simulink model "Simulink"  (R2025a)
settings: Solver=FixedStepDiscrete  StartTime=0.0  StopTime=80  FixedStep=1  RelTol=1e-3
libraries: simulink_extras x14
settings Model: SnapshotBufferSize=35  PacingRate=2  Creator=dell  LastModifiedBy=LENOVO

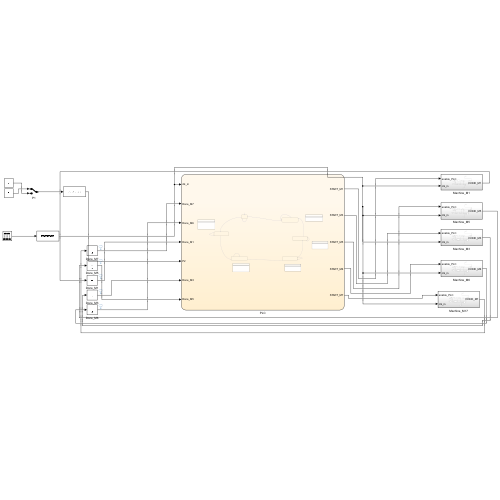
[thumbnail: Simulink's stored preview of the top-level diagram]
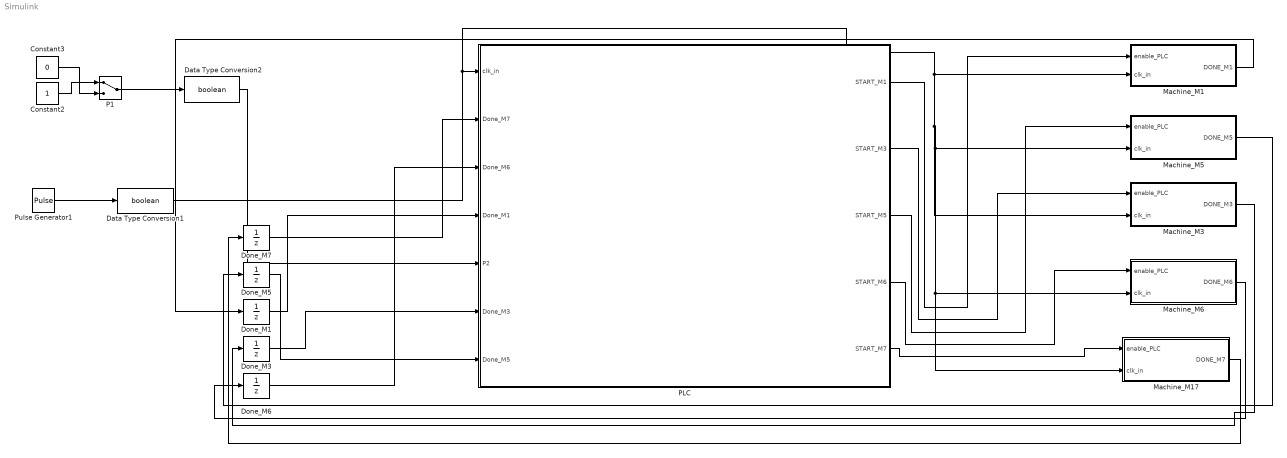
== system Simulink ==
  Constant2 : Constant  OutDataTypeStr=boolean
  Constant3 : Constant  Value=0  OutDataTypeStr=boolean
  Data Type Conversion1 : DataTypeConversion  OutDataTypeStr=boolean  SaturateOnIntegerOverflow=off  RndMeth=Floor
  Data Type Conversion2 : DataTypeConversion  OutDataTypeStr=boolean  SaturateOnIntegerOverflow=off  RndMeth=Floor
  Done_M{1,3,5..7} (5 alike) : UnitDelay  HasFrameUpgradeWarning=on
  Machine_M1 : Subsystem
  Machine_M17 : Subsystem
  Machine_M3 : Subsystem
  Machine_M5 : Subsystem
  Machine_M6 : Subsystem
  P1 : ManualSwitch
  PLC : Stateflow chart  TreatAsAtomicUnit=on
      settings: PortSchema="{\"entries\":[{\"content\":{\"sides\":[{\"content\":{\"connectorIds\":[\"In1\",\"In2\",\"In5\",\"In6\",\"In7\",\"In4\",\"In3\"]},\"type\":\"ConnectorPlacement.EquallySpacedRectSide\",\"uuid\":\"17f713a5-d983-479c-9e5e-6bf6c33331de\"},{\"content\":{\"connectorIds\":[\"Out1\",\"Out5\",\"Out2\",\"Out4\",\"Out3\"],\"side\":\"RIGHT\"},\"type\":\"ConnectorPlacement.EquallySpacedRectSide\",\"uuid\":\"d38a5cd9-5070-4c28-a52d-34bc8e7c4c10\"},{\"content\":{\"side\":\"TOP\"},\"type\":\"ConnectorPlacement.EquallySpacedRectSide\",\"uuid\":\"4971cf38-fc56-403e-81e2-f618dbc9148e\"}]},\"type\":\"ConnectorPlacement.EquallySpacedConnector\",\"uuid\":\"d5f3cc63-d87c-4b36-b9e3-2569f685359e\"}],\"packageUris\":[\"http://schema.mathworks.com/mf0/Connector/R2020b\"],\"version\":\"1.0\"}"
  Pulse Generator1 : DiscretePulseGenerator
  wires:
  Pulse Generator1/1 -> Data Type Conversion1/1
  Data Type Conversion1/1 -> Machine_M3/2(clk_in), Machine_M17/2(clk_in), Machine_M6/2(clk_in), Machine_M5/2(clk_in), Machine_M1/2(clk_in), PLC/1(clk_in)
  Constant3/1 -> P1/2
  Constant2/1 -> P1/1
  P1/1 -> Data Type Conversion2/1
  Done_M7/1 -> PLC/2(Done_M7)
  Done_M5/1 -> PLC/3(Done_M5)
  Done_M3/1 -> PLC/4(Done_M3)
  Done_M6/1 -> PLC/5(Done_M6)
  PLC/1(START_M1) -> Machine_M1/1(enable_PLC)
  PLC/2(START_M5) -> Machine_M5/1(enable_PLC)
  PLC/3(START_M7) -> Machine_M17/1(enable_PLC)
  PLC/4(START_M6) -> Machine_M6/1(enable_PLC)
  PLC/5(START_M3) -> Machine_M3/1(enable_PLC)
  Machine_M1/1(DONE_M1) -> Done_M1/1
  Machine_M5/1(DONE_M5) -> Done_M5/1
  Machine_M3/1(DONE_M3) -> Done_M3/1
  Machine_M6/1(DONE_M6) -> Done_M6/1
  Machine_M17/1(DONE_M7) -> Done_M7/1
  Done_M1/1 -> PLC/6(Done_M1)
  Data Type Conversion2/1 -> PLC/7(P2)

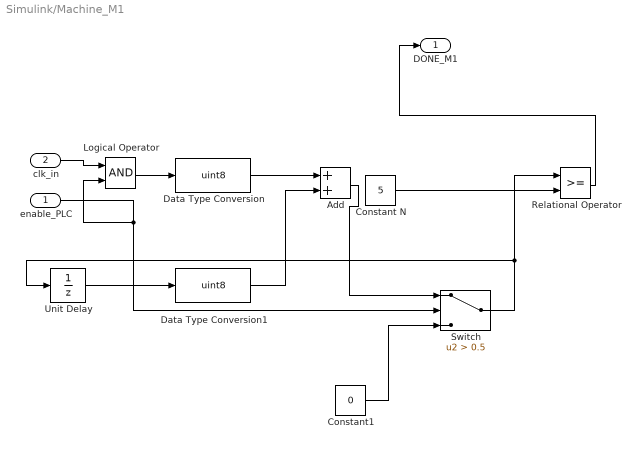
== system Simulink/Machine_M1 ==
  enable_PLC : Inport
  clk_in : Inport  Port=2
  Add : Sum
  Constant N : Constant  Value=5  OutDataTypeStr=uint8
  Constant1 : Constant  Value=0
  Data Type Conversion : DataTypeConversion  OutDataTypeStr=uint8  SaturateOnIntegerOverflow=off  RndMeth=Floor
  Data Type Conversion1 : DataTypeConversion  OutDataTypeStr=uint8  SaturateOnIntegerOverflow=off  RndMeth=Floor
  Logical Operator : Logic  AllPortsSameDT=off  OutDataTypeStr=boolean
  Relational Operator : RelationalOperator  OutDataTypeStr=boolean  RndMeth=Simplest  InputSameDT=off
  Switch : Switch  Criteria=u2 > Threshold  Threshold=0.5  SaturateOnIntegerOverflow=off  InputSameDT=off
  Unit Delay : UnitDelay  HasFrameUpgradeWarning=on
  DONE_M1 : Outport
  wires:
  Constant1/1 -> Switch/3
  Constant N/1 -> Relational Operator/2
  Relational Operator/1 -> DONE_M1/1
  clk_in/1 -> Logical Operator/1
  enable_PLC/1 -> Switch/2, Logical Operator/2
  Logical Operator/1 -> Data Type Conversion/1
  Unit Delay/1 -> Data Type Conversion1/1
  Add/1 -> Switch/1
  Switch/1 -> Relational Operator/1, Unit Delay/1
  Data Type Conversion/1 -> Add/1
  Data Type Conversion1/1 -> Add/2

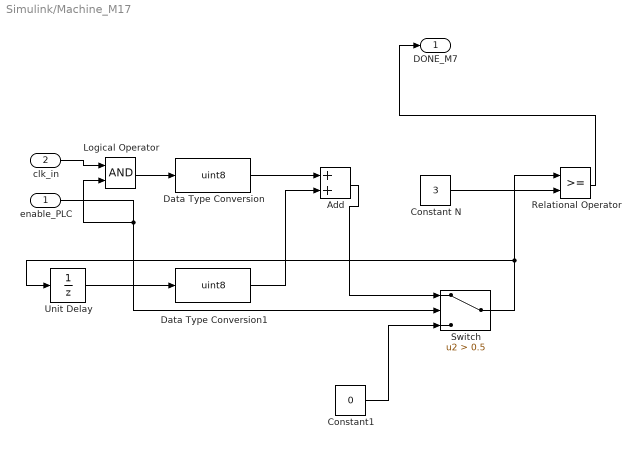
== system Simulink/Machine_M17 ==
  enable_PLC : Inport
  clk_in : Inport  Port=2
  Add : Sum
  Constant N : Constant  Value=3  OutDataTypeStr=uint8
  Constant1 : Constant  Value=0
  Data Type Conversion : DataTypeConversion  OutDataTypeStr=uint8  SaturateOnIntegerOverflow=off  RndMeth=Floor
  Data Type Conversion1 : DataTypeConversion  OutDataTypeStr=uint8  SaturateOnIntegerOverflow=off  RndMeth=Floor
  Logical Operator : Logic  AllPortsSameDT=off  OutDataTypeStr=boolean
  Relational Operator : RelationalOperator  OutDataTypeStr=boolean  RndMeth=Simplest  InputSameDT=off
  Switch : Switch  Criteria=u2 > Threshold  Threshold=0.5  SaturateOnIntegerOverflow=off  InputSameDT=off
  Unit Delay : UnitDelay  HasFrameUpgradeWarning=on
  DONE_M7 : Outport
  wires:
  Constant1/1 -> Switch/3
  Switch/1 -> Relational Operator/1, Unit Delay/1
  enable_PLC/1 -> Switch/2, Logical Operator/2
  Logical Operator/1 -> Data Type Conversion/1
  Constant N/1 -> Relational Operator/2
  clk_in/1 -> Logical Operator/1
  Data Type Conversion/1 -> Add/1
  Data Type Conversion1/1 -> Add/2
  Add/1 -> Switch/1
  Unit Delay/1 -> Data Type Conversion1/1
  Relational Operator/1 -> DONE_M7/1

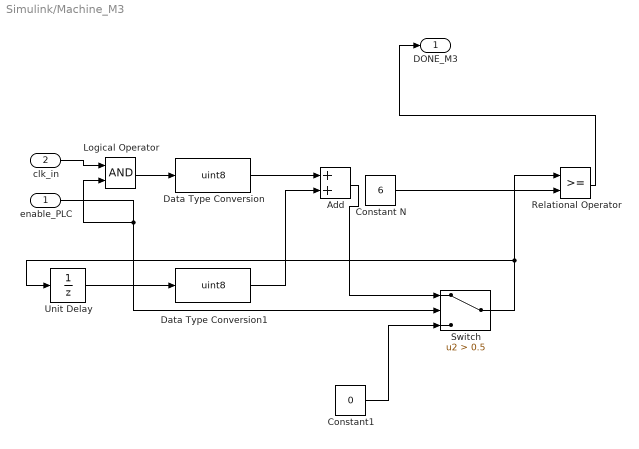
== system Simulink/Machine_M3 ==
  enable_PLC : Inport
  clk_in : Inport  Port=2
  Add : Sum
  Constant N : Constant  Value=6  OutDataTypeStr=uint8
  Constant1 : Constant  Value=0
  Data Type Conversion : DataTypeConversion  OutDataTypeStr=uint8  SaturateOnIntegerOverflow=off  RndMeth=Floor
  Data Type Conversion1 : DataTypeConversion  OutDataTypeStr=uint8  SaturateOnIntegerOverflow=off  RndMeth=Floor
  Logical Operator : Logic  AllPortsSameDT=off  OutDataTypeStr=boolean
  Relational Operator : RelationalOperator  OutDataTypeStr=boolean  RndMeth=Simplest  InputSameDT=off
  Switch : Switch  Criteria=u2 > Threshold  Threshold=0.5  SaturateOnIntegerOverflow=off  InputSameDT=off
  Unit Delay : UnitDelay  HasFrameUpgradeWarning=on
  DONE_M3 : Outport
  wires:
  Constant1/1 -> Switch/3
  Switch/1 -> Relational Operator/1, Unit Delay/1
  enable_PLC/1 -> Switch/2, Logical Operator/2
  Logical Operator/1 -> Data Type Conversion/1
  Constant N/1 -> Relational Operator/2
  clk_in/1 -> Logical Operator/1
  Data Type Conversion/1 -> Add/1
  Data Type Conversion1/1 -> Add/2
  Add/1 -> Switch/1
  Unit Delay/1 -> Data Type Conversion1/1
  Relational Operator/1 -> DONE_M3/1

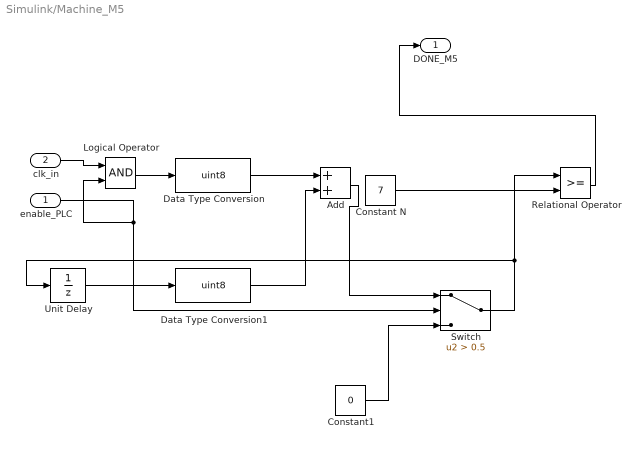
== system Simulink/Machine_M5 ==
  enable_PLC : Inport
  clk_in : Inport  Port=2
  Add : Sum
  Constant N : Constant  Value=7  OutDataTypeStr=uint8
  Constant1 : Constant  Value=0
  Data Type Conversion : DataTypeConversion  OutDataTypeStr=uint8  SaturateOnIntegerOverflow=off  RndMeth=Floor
  Data Type Conversion1 : DataTypeConversion  OutDataTypeStr=uint8  SaturateOnIntegerOverflow=off  RndMeth=Floor
  Logical Operator : Logic  AllPortsSameDT=off  OutDataTypeStr=boolean
  Relational Operator : RelationalOperator  OutDataTypeStr=boolean  RndMeth=Simplest  InputSameDT=off
  Switch : Switch  Criteria=u2 > Threshold  Threshold=0.5  SaturateOnIntegerOverflow=off  InputSameDT=off
  Unit Delay : UnitDelay  HasFrameUpgradeWarning=on
  DONE_M5 : Outport
  wires:
  Constant1/1 -> Switch/3
  Switch/1 -> Relational Operator/1, Unit Delay/1
  enable_PLC/1 -> Switch/2, Logical Operator/2
  Logical Operator/1 -> Data Type Conversion/1
  Constant N/1 -> Relational Operator/2
  clk_in/1 -> Logical Operator/1
  Data Type Conversion/1 -> Add/1
  Data Type Conversion1/1 -> Add/2
  Add/1 -> Switch/1
  Unit Delay/1 -> Data Type Conversion1/1
  Relational Operator/1 -> DONE_M5/1

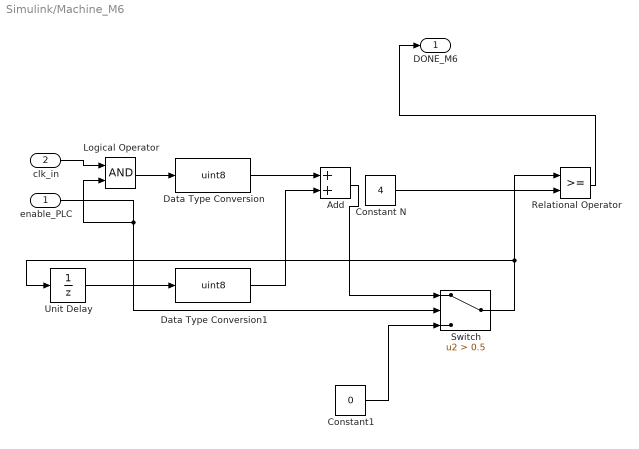
== system Simulink/Machine_M6 ==
  enable_PLC : Inport
  clk_in : Inport  Port=2
  Add : Sum
  Constant N : Constant  Value=4  OutDataTypeStr=uint8
  Constant1 : Constant  Value=0
  Data Type Conversion : DataTypeConversion  OutDataTypeStr=uint8  SaturateOnIntegerOverflow=off  RndMeth=Floor
  Data Type Conversion1 : DataTypeConversion  OutDataTypeStr=uint8  SaturateOnIntegerOverflow=off  RndMeth=Floor
  Logical Operator : Logic  AllPortsSameDT=off  OutDataTypeStr=boolean
  Relational Operator : RelationalOperator  OutDataTypeStr=boolean  RndMeth=Simplest  InputSameDT=off
  Switch : Switch  Criteria=u2 > Threshold  Threshold=0.5  SaturateOnIntegerOverflow=off  InputSameDT=off
  Unit Delay : UnitDelay  HasFrameUpgradeWarning=on
  DONE_M6 : Outport
  wires:
  Constant1/1 -> Switch/3
  Switch/1 -> Relational Operator/1, Unit Delay/1
  enable_PLC/1 -> Switch/2, Logical Operator/2
  Logical Operator/1 -> Data Type Conversion/1
  Constant N/1 -> Relational Operator/2
  clk_in/1 -> Logical Operator/1
  Data Type Conversion/1 -> Add/1
  Data Type Conversion1/1 -> Add/2
  Add/1 -> Switch/1
  Unit Delay/1 -> Data Type Conversion1/1
  Relational Operator/1 -> DONE_M6/1

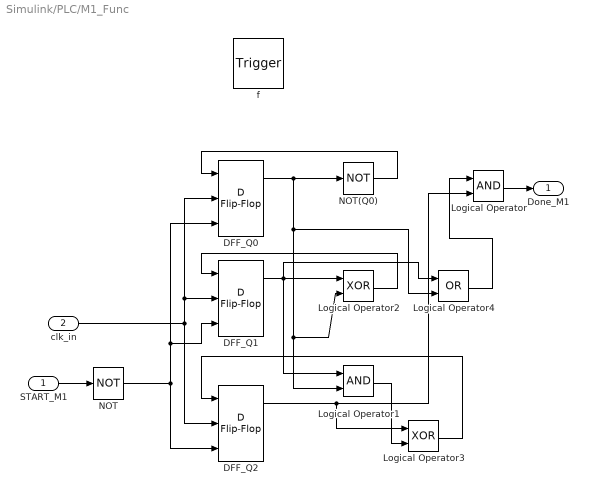
== system Simulink/PLC/M1_Func ==
  START_M1 : Inport  OutDataTypeStr=double  PortDimensions=1
  clk_in : Inport  Port=2  OutDataTypeStr=double  PortDimensions=1
  f : TriggerPort  TriggerType=function-call  VariantControl=(inherit)
      settings: CopyFcn=Stateflow.SLINSF.SimulinkMan.removeBlockPreDeleteFcn  PreDeleteFcn=Stateflow.SLINSF.SimulinkMan.unsafePredeleteFcn
  DFF_Q0 : simulink_extras/Flip Flops/D Flip-Flop
  DFF_Q1 : simulink_extras/Flip Flops/D Flip-Flop
  DFF_Q2 : simulink_extras/Flip Flops/D Flip-Flop
  Logical Operator : Logic  AllPortsSameDT=off  OutDataTypeStr=boolean
  Logical Operator1 : Logic  AllPortsSameDT=off  OutDataTypeStr=boolean
  Logical Operator2 : Logic  Operator=XOR  AllPortsSameDT=off  OutDataTypeStr=boolean
  Logical Operator3 : Logic  Operator=XOR  AllPortsSameDT=off  OutDataTypeStr=boolean
  Logical Operator4 : Logic  Operator=OR  AllPortsSameDT=off  OutDataTypeStr=boolean
  NOT : Logic  Operator=NOT  IconShape=distinctive  AllPortsSameDT=off  OutDataTypeStr=boolean
  NOT(Q0) : Logic  Operator=NOT  IconShape=distinctive  AllPortsSameDT=off  OutDataTypeStr=boolean
  Done_M1 : Outport  OutDataTypeStr=boolean  PortDimensions=1
  wires:
  START_M1/1 -> NOT/1
  NOT/1 -> DFF_Q0/3, DFF_Q1/3, DFF_Q2/3
  clk_in/1 -> DFF_Q0/2, DFF_Q1/2, DFF_Q2/2
  DFF_Q0/1 -> Logical Operator4/2, Logical Operator1/2, Logical Operator2/2, NOT(Q0)/1
  DFF_Q1/1 -> Logical Operator4/1, Logical Operator1/1, Logical Operator2/1
  DFF_Q2/1 -> Logical Operator/2, Logical Operator3/1
  Logical Operator1/1 -> Logical Operator3/2
  NOT(Q0)/1 -> DFF_Q0/1
  Logical Operator2/1 -> DFF_Q1/1
  Logical Operator3/1 -> DFF_Q2/1
  Logical Operator/1 -> Done_M1/1
  Logical Operator4/1 -> Logical Operator/1

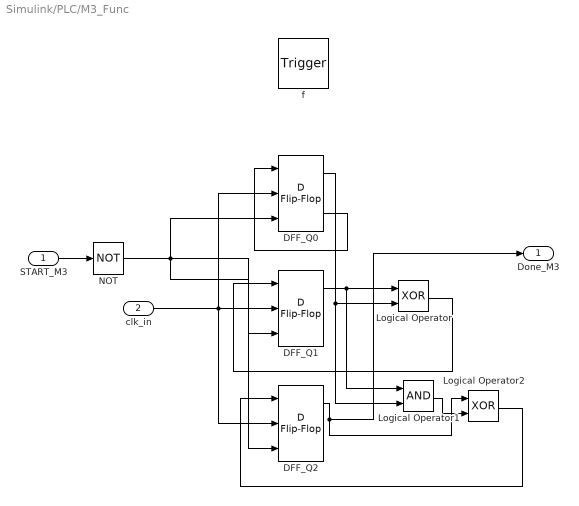
== system Simulink/PLC/M3_Func ==
  START_M3 : Inport  OutDataTypeStr=boolean  PortDimensions=1
  clk_in : Inport  Port=2  OutDataTypeStr=boolean  PortDimensions=1
  f : TriggerPort  TriggerType=function-call  VariantControl=(inherit)
      settings: CopyFcn=Stateflow.SLINSF.SimulinkMan.removeBlockPreDeleteFcn  PreDeleteFcn=Stateflow.SLINSF.SimulinkMan.unsafePredeleteFcn
  DFF_Q0 : simulink_extras/Flip Flops/D Flip-Flop
  DFF_Q1 : simulink_extras/Flip Flops/D Flip-Flop
  DFF_Q2 : simulink_extras/Flip Flops/D Flip-Flop
  Logical Operator : Logic  Operator=XOR  AllPortsSameDT=off  OutDataTypeStr=boolean
  Logical Operator1 : Logic  AllPortsSameDT=off  OutDataTypeStr=boolean
  Logical Operator2 : Logic  Operator=XOR  AllPortsSameDT=off  OutDataTypeStr=boolean
  NOT : Logic  Operator=NOT  IconShape=distinctive  AllPortsSameDT=off  OutDataTypeStr=boolean
  Done_M3 : Outport  OutDataTypeStr=boolean  PortDimensions=1
  wires:
  clk_in/1 -> DFF_Q2/2, DFF_Q1/2, DFF_Q0/2
  START_M3/1 -> NOT/1
  NOT/1 -> DFF_Q2/3, DFF_Q1/3, DFF_Q0/3
  DFF_Q0/2 -> DFF_Q0/1
  DFF_Q1/1 -> Logical Operator1/1, Logical Operator/1
  DFF_Q0/1 -> Logical Operator1/2, Logical Operator/2
  Logical Operator/1 -> DFF_Q1/1
  DFF_Q2/1 -> Done_M3/1, Logical Operator2/1
  Logical Operator1/1 -> Logical Operator2/2
  Logical Operator2/1 -> DFF_Q2/1

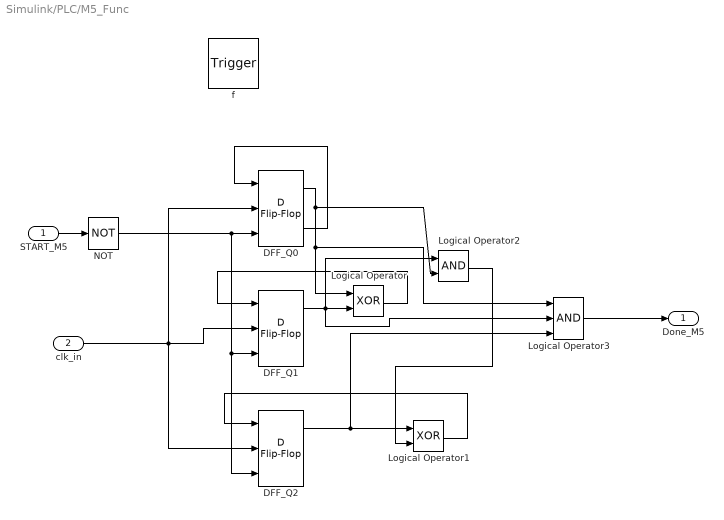
== system Simulink/PLC/M5_Func ==
  START_M5 : Inport  OutDataTypeStr=boolean  PortDimensions=1
  clk_in : Inport  Port=2  OutDataTypeStr=boolean  PortDimensions=1
  f : TriggerPort  TriggerType=function-call  VariantControl=(inherit)
      settings: CopyFcn=Stateflow.SLINSF.SimulinkMan.removeBlockPreDeleteFcn  PreDeleteFcn=Stateflow.SLINSF.SimulinkMan.unsafePredeleteFcn
  DFF_Q0 : simulink_extras/Flip Flops/D Flip-Flop
  DFF_Q1 : simulink_extras/Flip Flops/D Flip-Flop
  DFF_Q2 : simulink_extras/Flip Flops/D Flip-Flop
  Logical Operator : Logic  Operator=XOR  AllPortsSameDT=off  OutDataTypeStr=boolean
  Logical Operator1 : Logic  Operator=XOR  AllPortsSameDT=off  OutDataTypeStr=boolean
  Logical Operator2 : Logic  AllPortsSameDT=off  OutDataTypeStr=boolean
  Logical Operator3 : Logic  Inputs=3  AllPortsSameDT=off  OutDataTypeStr=boolean
  NOT : Logic  Operator=NOT  IconShape=distinctive  AllPortsSameDT=off  OutDataTypeStr=boolean
  Done_M5 : Outport  OutDataTypeStr=boolean  PortDimensions=1
  wires:
  clk_in/1 -> DFF_Q2/2, DFF_Q0/2, DFF_Q1/2
  START_M5/1 -> NOT/1
  NOT/1 -> DFF_Q2/3, DFF_Q1/3, DFF_Q0/3
  DFF_Q0/2 -> DFF_Q0/1
  DFF_Q1/1 -> Logical Operator3/2, Logical Operator2/1, Logical Operator/2
  DFF_Q0/1 -> Logical Operator2/2, Logical Operator3/1, Logical Operator/1
  Logical Operator/1 -> DFF_Q1/1
  Logical Operator2/1 -> Logical Operator1/2
  DFF_Q2/1 -> Logical Operator3/3, Logical Operator1/1
  Logical Operator1/1 -> DFF_Q2/1
  Logical Operator3/1 -> Done_M5/1

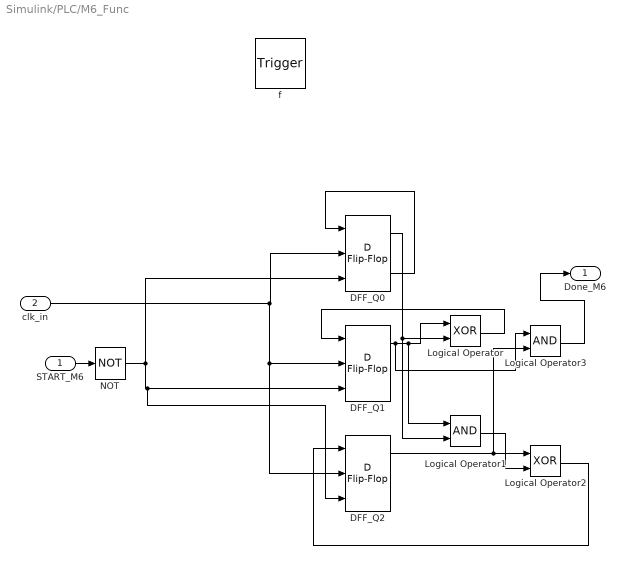
== system Simulink/PLC/M6_Func ==
  START_M6 : Inport  OutDataTypeStr=boolean  PortDimensions=1
  clk_in : Inport  Port=2  OutDataTypeStr=boolean  PortDimensions=1
  f : TriggerPort  TriggerType=function-call  VariantControl=(inherit)
      settings: CopyFcn=Stateflow.SLINSF.SimulinkMan.removeBlockPreDeleteFcn  PreDeleteFcn=Stateflow.SLINSF.SimulinkMan.unsafePredeleteFcn
  DFF_Q0 : simulink_extras/Flip Flops/D Flip-Flop
  DFF_Q1 : simulink_extras/Flip Flops/D Flip-Flop
  DFF_Q2 : simulink_extras/Flip Flops/D Flip-Flop
  Logical Operator : Logic  Operator=XOR  AllPortsSameDT=off  OutDataTypeStr=boolean
  Logical Operator1 : Logic  AllPortsSameDT=off  OutDataTypeStr=boolean
  Logical Operator2 : Logic  Operator=XOR  AllPortsSameDT=off  OutDataTypeStr=boolean
  Logical Operator3 : Logic  AllPortsSameDT=off  OutDataTypeStr=boolean
  NOT : Logic  Operator=NOT  IconShape=distinctive  AllPortsSameDT=off  OutDataTypeStr=boolean
  Done_M6 : Outport  OutDataTypeStr=boolean  PortDimensions=1
  wires:
  clk_in/1 -> DFF_Q2/2, DFF_Q1/2, DFF_Q0/2
  START_M6/1 -> NOT/1
  NOT/1 -> DFF_Q0/3, DFF_Q2/3, DFF_Q1/3
  DFF_Q0/2 -> DFF_Q0/1
  DFF_Q1/1 -> Logical Operator3/1, Logical Operator1/1, Logical Operator/1
  DFF_Q0/1 -> Logical Operator1/2, Logical Operator/2
  Logical Operator/1 -> DFF_Q1/1
  Logical Operator1/1 -> Logical Operator2/2
  DFF_Q2/1 -> Logical Operator3/2, Logical Operator2/1
  Logical Operator2/1 -> DFF_Q2/1
  Logical Operator3/1 -> Done_M6/1

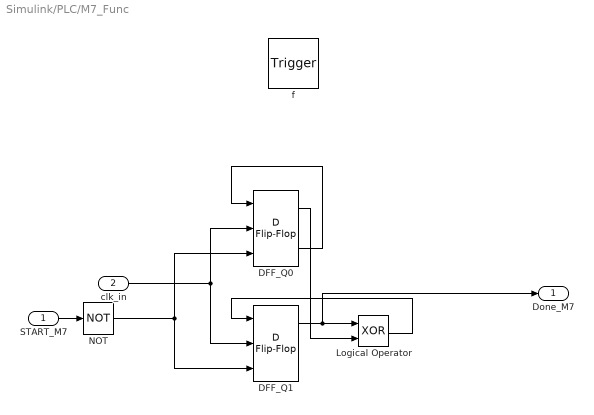
== system Simulink/PLC/M7_Func ==
  START_M7 : Inport  OutDataTypeStr=boolean  PortDimensions=1
  clk_in : Inport  Port=2  OutDataTypeStr=boolean  PortDimensions=1
  f : TriggerPort  TriggerType=function-call  VariantControl=(inherit)
      settings: CopyFcn=Stateflow.SLINSF.SimulinkMan.removeBlockPreDeleteFcn  PreDeleteFcn=Stateflow.SLINSF.SimulinkMan.unsafePredeleteFcn
  DFF_Q0 : simulink_extras/Flip Flops/D Flip-Flop
  DFF_Q1 : simulink_extras/Flip Flops/D Flip-Flop
  Logical Operator : Logic  Operator=XOR  AllPortsSameDT=off  OutDataTypeStr=boolean
  NOT : Logic  Operator=NOT  IconShape=distinctive  AllPortsSameDT=off  OutDataTypeStr=boolean
  Done_M7 : Outport  OutDataTypeStr=boolean  PortDimensions=1
  wires:
  clk_in/1 -> DFF_Q0/2, DFF_Q1/2
  START_M7/1 -> NOT/1
  NOT/1 -> DFF_Q0/3, DFF_Q1/3
  DFF_Q0/2 -> DFF_Q0/1
  DFF_Q1/1 -> Done_M7/1, Logical Operator/1
  DFF_Q0/1 -> Logical Operator/2
  Logical Operator/1 -> DFF_Q1/1

== stateflow chart Simulink/PLC ==
  settings: sampleTime=2
  state IDLE
  state Done_M7 = M7_Func(START_M7,clk_in) [function]
  state M7
    START_M7=true;
  state Done_M1 = M1_Func(START_M1,clk_in) [function]
  state M1
    START_M1=true;
  state M6
    START_M6= true;
  state Done_M6 = M6_Func(START_M6,clk_in) [function]
  state M5
    START_M5=true;
  state M3
    START_M3=true;
  state Done_M5 = M5_Func(START_M5,clk_in) [function]
  state Done_M3 = M3_Func(START_M3,clk_in) [function]
  (default) -> IDLE
  M7 -> M7 [order 1] : [Done_M7==0]
  M7 -> IDLE [order 2] : [Done_M7==1]
  IDLE -> M1 [order 1] : [P2==1]
  M6 -> M7 [order 1] : [Done_M6==1]
  IDLE -> IDLE [order 2] : [P2==0]
  M1 -> M1 [order 2] : [Done_M1==0]
  M1 -> M5 [order 1] : [Done_M1==1]
  M6 -> M6 [order 2] : [Done_M6==0]
  M3 -> M6 [order 1] : [Done_M3==1]
  M5 -> M5 [order 2] : [Done_M5==0]
  M3 -> M3 [order 2] : [Done_M3==0]
  M5 -> M3 [order 1] : [Done_M5==1]
  data: START_M7 function_input boolean size=1; Done_M7 function_output boolean size=1; clk_in function_input boolean size=1; Done_M1 function_output boolean size=1; START_M1 function_input double size=1; clk_in function_input double size=1; START_M6 function_input boolean size=1; Done_M6 function_output boolean size=1; clk_in function_input boolean size=1; START_M5 function_input boolean size=1; Done_M5 function_output boolean size=1; clk_in function_input boolean size=1; START_M3 function_input boolean size=1; Done_M3 function_output boolean size=1; clk_in function_input boolean size=1; clk_in input; START_M1 output boolean size=1; START_M5 output boolean size=1; START_M7 output boolean size=1; START_M6 output boolean size=1; START_M3 output boolean size=1; Done_M7 input boolean size=1; Done_M5 input boolean size=1; Done_M3 input boolean size=1; Done_M6 input boolean size=1; Done_M1 input boolean size=1; P2 input
